simulink model "current_phasor_commutation"  (R2016a)
settings: Solver=ode23t  StartTime=0.0  StopTime=1  MaxStep=1e-4  RelTol=1e-4  AbsTol=1e-4
undefined symbols (not defined in the file): j, P
libraries: fl_lib x8, nesl_utility x8, pe_lib x3, ThreePhaseExamples_lib x1
Description:
  | Three-Phase Custom PMSM
  | 
  | This example shows a custom Simscape(TM) implementation of
  | a Permanent Magnet Synchronous Machine (PMSM). To view the
  | PMSM source code, double-click on the motor block and then
  | click on the hyperlink 'Source code'. This test circuit shows the
  | PMSM being used as a generator, the rectifier block converting
  | the induced AC back EMFs to a DC voltage which is in turn
  | applied to a resistive load.
  | 
  | 
  | 
  | Copyright 2008-2016 The MathWorks, Inc.
settings Model: Creator=MathWorks  LastModifiedBy=hbjo
settings DataIOCC: LimitDataPoints=on  SaveFormat=Array
settings DebuggingCC: UnderspecifiedInitializationDetection=Classic  MergeDetectMultiDrivingBlocksExec=none
settings HardwareCC: ProdBitPerPointer=32  ProdLargestAtomicFloat=None  ProdIntDivRoundTo=Undefined  ProdEndianess=Unspecified  ProdWordSize=32  ProdHWDeviceType=32-bit Generic
settings ModelReferenceCC: PropagateSignalLabelsOutOfModel=off
settings ConfigComp: CovModelRefEnable=Off  CovSFcnEnable=off
settings SimscapeCC: SimscapeLogDataHistory=50000

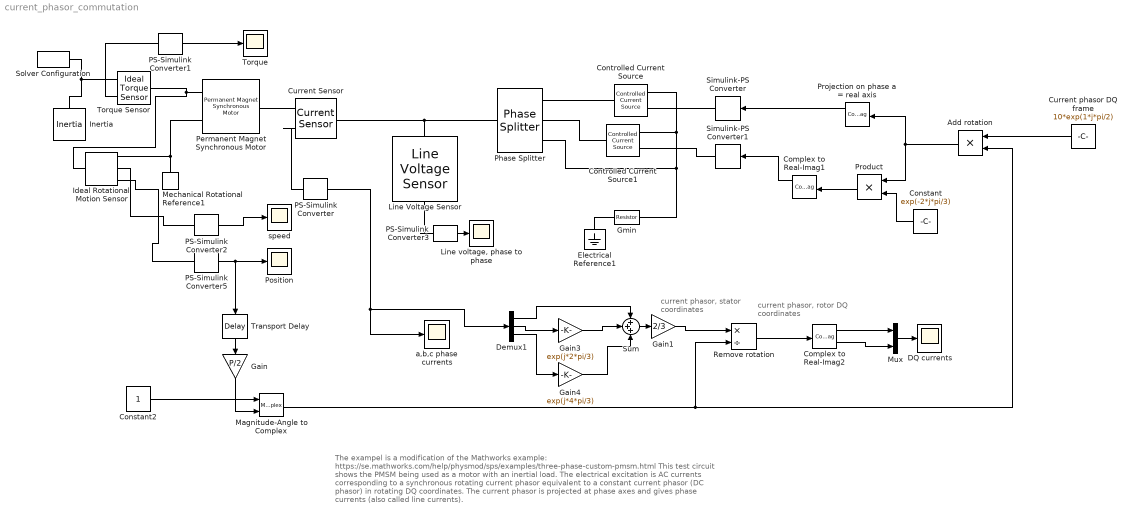
== system current_phasor_commutation ==
  note: current phasor,
      |  stator coordinates
  note: current phasor,
      | rotor DQ coordinates
  note: The exampel is a modification of the Mathworks example: https://se.mathworks.com/help/physmod/sps/examples/three-phase-custom-pmsm.html
      | This test circuit shows the PMSM being used as a motor with an inertial load.
      | The electrical excitation is AC currents corresponding to a synchronous rotating current phasor
      | equivalent to a constant current phasor (DC phasor) in rotating DQ coordinates.
      | The current phasor is projected at phase axes and gives phase currents (also called line currents).
  Add rotation : Product
  Complex to Real-Imag1 : ComplexToRealImag
  Complex to Real-Imag2 : ComplexToRealImag
  Constant : Constant  Value=exp(-2*j*pi/3)
  Constant2 : Constant
  Controlled Current Source : fl_lib/Electrical/Electrical Sources/Controlled Current Source
  Controlled Current Source1 : fl_lib/Electrical/Electrical Sources/Controlled Current Source
  Current Sensor : pe_lib/Sensors/Current Sensor
  Current phasor DQ frame : Constant  Value=10*exp(1*j*pi/2)
  DQ currents : Scope
  Demux1 : Demux  Outputs=3
  Electrical Reference1 : fl_lib/Electrical/Electrical Elements/Electrical Reference
  Gain : Gain  Gain=P/2
  Gain1 : Gain  Gain=2/3
  Gain3 : Gain  Gain=exp(j*2*pi/3)
  Gain4 : Gain  Gain=exp(j*4*pi/3)
  Gmin : fl_lib/Electrical/Electrical Elements/Resistor  R=1e9 Ohm  i_specify=off  i_priority=High  i=0 A  v_specify=off  v_priority=High  v=0 V
  Ideal Rotational Motion Sensor : fl_lib/Mechanical/Mechanical Sensors/Ideal Rotational Motion Sensor  offset=0 rad
  Inertia : fl_lib/Mechanical/Rotational Elements/Inertia  inertia=J kg*m^2  w_specify=off  w_priority=High  w=0 rad/s  t_specify=off  t_priority=None  t=0 N*m
  Line Voltage Sensor : pe_lib/Sensors/Line Voltage Sensor
  "Line voltage, phase to phase" : Scope
  Magnitude-Angle to Complex : MagnitudeAngleToComplex
  Mechanical Rotational Reference1 : fl_lib/Mechanical/Rotational Elements/Mechanical Rotational Reference
  Mux : Mux  Inputs=2
  PS-Simulink Converter : nesl_utility/PS-Simulink Converter  PhysicalDomain=network_engine_domain  SubClassName=ps_output  LeftPortType=input  RightPortType=output  PseudoPeriodic=off  Frequencies=[]  Unit=A  AffineConversion=off
  PS-Simulink Converter1 : nesl_utility/PS-Simulink Converter  PhysicalDomain=network_engine_domain  SubClassName=ps_output  LeftPortType=input  RightPortType=output  PseudoPeriodic=off  Frequencies=[]  Unit=N*m  AffineConversion=off
  PS-Simulink Converter2 : nesl_utility/PS-Simulink Converter  PhysicalDomain=network_engine_domain  SubClassName=ps_output  LeftPortType=input  RightPortType=output  PseudoPeriodic=off  Frequencies=[]  Unit=rad/s  AffineConversion=off
  PS-Simulink Converter3 : nesl_utility/PS-Simulink Converter  PhysicalDomain=network_engine_domain  SubClassName=ps_output  LeftPortType=input  RightPortType=output  PseudoPeriodic=off  Frequencies=[]  Unit=V  AffineConversion=off
  PS-Simulink Converter5 : nesl_utility/PS-Simulink Converter  PhysicalDomain=network_engine_domain  SubClassName=ps_output  LeftPortType=input  RightPortType=output  PseudoPeriodic=off  Frequencies=[]  Unit=rad  AffineConversion=off
  Permanent Magnet Synchronous Motor : ThreePhaseExamples_lib/Permanent Magnet Synchronous Motor  nPolePairs=P/2  pm_flux_linkage=psi Wb  Ld=L H  Lq=L H  Rs=R Ohm  wNominal=0 rad/s  angular_position_diff_specify=off  angular_position_diff_priority=None  angular_position_diff=0 rad  i_d_specify=off  i_d_priority=High  i_d=0 A  i_q_specify=off  i_q_priority=High  i_q=0 A
  Phase Splitter : pe_lib/Connections/Phase Splitter
  Position : Scope
  Product : Product
  Projection on phase a = real axis : ComplexToRealImag
  Remove rotation : Product  Inputs=*/
  Simulink-PS Converter : nesl_utility/Simulink-PS Converter  PhysicalDomain=network_engine_domain  SubClassName=ps_input  LeftPortType=input  RightPortType=output  PseudoPeriodic=off  Frequencies=[]  NoiseDistribution=none  NoiseParameters=[]  Unit=A  AffineConversion=off  InputFiltering=off  SimscapeFilterOrder=1  InputFilterTimeConstant=0.001  UdotUserProvided=1
  Simulink-PS Converter1 : nesl_utility/Simulink-PS Converter  PhysicalDomain=network_engine_domain  SubClassName=ps_input  LeftPortType=input  RightPortType=output  PseudoPeriodic=off  Frequencies=[]  NoiseDistribution=none  NoiseParameters=[]  Unit=A  AffineConversion=off  InputFiltering=off  SimscapeFilterOrder=1  InputFilterTimeConstant=0.001  UdotUserProvided=1
  Solver Configuration : nesl_utility/Solver Configuration  PhysicalDomain=network_engine_domain  SubClassName=solver  LeftPortType=input  RightPortType=generic  Accelerate=off  Tones=[]  Harmonics=[]  SimulateNoise=off  Profile=off  UseLocalSampling=off  EnableSwitchedLinearOptims=on  FrequencyDomain=off  UseCCode=off  RelTol=0.001  AbsTol=1e-06  MinStep=1e-09  ToWorkspace=off  RevertToSquareIcSolve=off  NumHomotopyIterations=100  PhasorMode=off  PhasorModeNumHarmonics=1  OverrideAbsTol=off  DoDC=off  ResidualTolerance=1e-9  UseLocalSolver=on  LocalSolverChoice=NE_BACKWARD_EULER_ADVANCER  LocalSolverSampleTime=1e-5  DoFixedCost=on  MaxNonlinIter=3  MaxModeIter=2  LinearAlgebra=Sparse  DelaysMemoryBudget=1024  AutomaticFiltering=on  FilteringTimeConstant=0.001
  Sum : Sum  Inputs=+++
  Torque : Scope
  Torque Sensor : fl_lib/Mechanical/Mechanical Sensors/Ideal Torque Sensor
  Transport Delay : TransportDelay  DelayTime=1e-5
  a,b,c phase currents : Scope
  speed : Scope
  wires:
  PS-Simulink Converter1/1 -> Torque/1
  PS-Simulink Converter3/1 -> "Line voltage, phase to phase"/1
  PS-Simulink Converter2/1 -> speed/1
  PS-Simulink Converter5/1 -> Transport Delay/1, Position/1
  Complex to Real-Imag1/1 -> Simulink-PS Converter1/1
  Projection on phase a = real axis/1 -> Simulink-PS Converter/1
  Constant/1 -> Product/2
  Product/1 -> Complex to Real-Imag1/1
  Add rotation/1 -> Projection on phase a = real axis/1, Product/1
  Constant2/1 -> Magnitude-Angle to Complex/1
  Current phasor DQ frame/1 -> Add rotation/1
  Transport Delay/1 -> Gain/1
  Magnitude-Angle to Complex/1 -> Remove rotation/2, Add rotation/2
  Gain/1 -> Magnitude-Angle to Complex/2
  Demux1/2 -> Gain3/1
  Demux1/3 -> Gain4/1
  Gain3/1 -> Sum/2
  Demux1/1 -> Sum/1
  Gain4/1 -> Sum/3
  Remove rotation/1 -> Complex to Real-Imag2/1
  Mux/1 -> DQ currents/1
  Complex to Real-Imag2/1 -> Mux/1
  Complex to Real-Imag2/2 -> Mux/2
  PS-Simulink Converter/1 -> Demux1/1, a,b,c phase currents/1
  Sum/1 -> Gain1/1
  Gain1/1 -> Remove rotation/1
  connections:
  Permanent Magnet Synchronous Motor/RConn2 -- Ideal Rotational Motion Sensor/RConn1 -- Mechanical Rotational Reference1/LConn1
  Current Sensor/RConn1 -- PS-Simulink Converter/LConn1
  Ideal Rotational Motion Sensor/LConn1 -- Torque Sensor/LConn1 -- Permanent Magnet Synchronous Motor/RConn1
  Inertia/LConn1 -- Torque Sensor/RConn1 -- Solver Configuration/RConn1
  Electrical Reference1/LConn1 -- Gmin/LConn1
  PS-Simulink Converter3/LConn1 -- Line Voltage Sensor/RConn1
  Torque Sensor/RConn2 -- PS-Simulink Converter1/LConn1
  Phase Splitter/LConn1 -- Line Voltage Sensor/LConn1 -- Current Sensor/LConn1
  Controlled Current Source/LConn1 -- Phase Splitter/RConn1
  PS-Simulink Converter2/LConn1 -- Ideal Rotational Motion Sensor/RConn2
  PS-Simulink Converter5/LConn1 -- Ideal Rotational Motion Sensor/RConn3
  Controlled Current Source/RConn1 -- Simulink-PS Converter/RConn1
  Controlled Current Source1/RConn1 -- Simulink-PS Converter1/RConn1
  Phase Splitter/RConn3 -- Gmin/RConn1 -- Controlled Current Source/RConn2 -- Controlled Current Source1/RConn2
  Controlled Current Source1/LConn1 -- Phase Splitter/RConn2
  Current Sensor/RConn2 -- Permanent Magnet Synchronous Motor/LConn1
